simulink model "test_p"  (R2022a)
settings: Solver=FixedStepAuto  StartTime=0.0  StopTime=20  FixedStep=0.005  RelTol=1e-3
values from neighbouring files (symbols this model uses):
  AttDyna_Ixx = 0.0211    [InitParameters.m]
  AttDyna_Iyy = 0.0219    [InitParameters.m]
  AttDyna_Izz = 0.0366    [InitParameters.m]
  ConEfficiency_drone_cM = 1.779e-07    [InitParameters.m]
  ConEfficiency_drone_cT = 1.105e-05    [InitParameters.m]
  ConEfficiency_drone_R = 0.225    [InitParameters.m]
  PowerUnit_CR = 1148    [InitParameters.m]
  PowerUnit_Tm = 0.02    [InitParameters.m]
  PowerUnit_wb = -141.4    [InitParameters.m]
libraries: simulink x53, slpidlib x15, fuzblock x12, mpclib x1
(part 1 of 3)
settings Model: Creator=ZhangZheng  LastModifiedBy=Administrator
settings SolverCC: AlgebraicLoopSolver=TrustRegion
settings DataIOCC: ReturnWorkspaceOutputs=off
settings DebuggingCC: UnconnectedInputMsg=warning  UnconnectedOutputMsg=warning  UnconnectedLineMsg=warning  SFMachineParentedDataDiag=warning  ArithmeticOperatorsInVariantConditions=warning
settings SFSimCC: SimUseLocalCustomCode=off  CustomCodeUndefinedFunction=UseInterfaceOnly
settings RTWCC: RTWUseLocalCustomCode=off

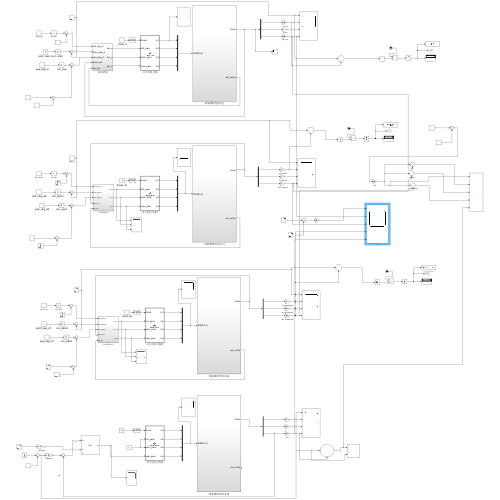
[thumbnail: Simulink's stored preview of the top-level diagram]
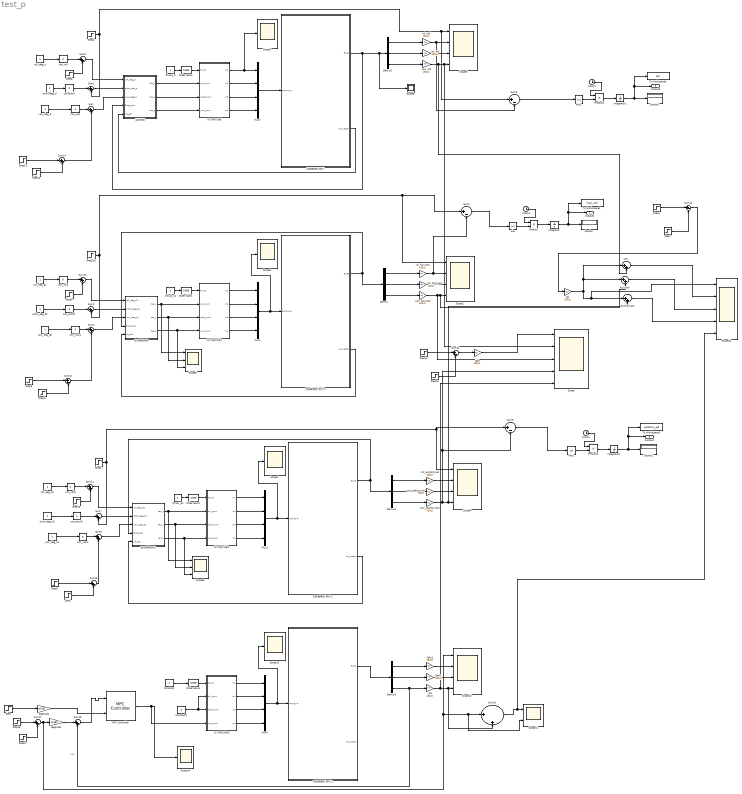
== system test_p ==
  note: sun
  Abs : Abs  SaturateOnIntegerOverflow=off
  Abs1 : Abs  SaturateOnIntegerOverflow=off
  Abs2 : Abs  SaturateOnIntegerOverflow=off
  Clock1 : Clock
      settings: Decimation=20
  Clock2 : Clock
      settings: Decimation=20
  Clock4 : Clock
      settings: Decimation=20
  Constant : Constant
  Constant1 : Constant  Value=0
  Demux{,1..3} (4 alike) : Demux  Outputs=3
  Display : Display
  Display1 : Display
  Display2 : Display
  Gain : Gain  Gain=180/pi
  Gain1 : Gain  Gain=180/pi
  Gain3 : Gain  Gain=180/pi
  Integrator : Integrator
  Integrator1 : Integrator
  Integrator2 : Integrator
  MPC Controller : mpclib/MPC Controller  SCDEnableBlockLinearizationSpecification=on  mpcobj=mpc1  is_multiple=0  enable_value=0  return_u0=off  updateMPCinCallerWorkspace=on  md_inport=off  mv_inport=off  uref_inport=off  return_cost=off  return_mvseq=off  return_qpstatus=off  return_xseq=off  return_state=off  return_ovseq=off  state_inport=off  umin_inport=off  umax_inport=off  ymin_inport=off  ymax_inport=off  cc_inport=off  ywt_inport=off  uwt_inport=off  duwt_inport=off  rhoeps_inport=off  pm_inport=off  MaximumP=10  HorizonChoice=FixedHorizon  n_ts=0.01  n_p=10  n_mv=1  n_md=0  n_ud=0  n_mo=1  n_uo=0  BlockDataType=double  SampleTimeInherited=off  switch_inport=off
  Mux{1..4} (4 alike) : Mux
  Product : Product
  Product1 : Product
  Product2 : Product
  Scope : Scope  NumInputPorts=5
  Scope{1,4,6,12} (4 alike) : Scope  NumInputPorts=4
  Scope10 : Scope  NumInputPorts=5
  Scope11 : Scope  NumInputPorts=2
  Scope{2..3,7,9,13..14} (6 alike) : Scope
  Scope5 : Scope  NumInputPorts=3
  Scope8 : Scope  NumInputPorts=3
  Slider Gain{1..4} (4 alike) : simulink/Math Operations/Slider Gain  gain=0.609  low=0  high=1
  Step : Step  Time=0  After=0  SampleTime=0
  Step1 : Step  Time=8  After=0  SampleTime=0
  Step{2..3,5..6,8..10,13} (8 alike) : Step  Time=5  After=0  SampleTime=0
  Step11 : Step  Time=8  After=0  SampleTime=0
  Step12 : Step  Time=8  After=0  SampleTime=0
  Step14 : Step  Time=5  After=0.05  SampleTime=0
  Step15 : Step  Time=6  After=0.05  SampleTime=0
  Step16 : Step  Time=5  After=2.866  SampleTime=0
  Step17 : Step  Time=6  After=2.866  SampleTime=0
  Step4 : Step  Time=5  After=0.05  SampleTime=0
  Step7 : Step  Time=6  After=0.05  SampleTime=0
  Step_pit : Step  Time=5  After=0  SampleTime=0
  Sum{,1..3,6..7,9..11,18..19} (11 alike) : Sum  Inputs=|++
  Sum{4..5,8,12..17} (9 alike) : Sum  Inputs=|+-
  To Workspace1 : ToWorkspace  VariableName=fuzzy_pid  SaveFormat=Timeseries  SampleTime=-1
  To Workspace2 : ToWorkspace  VariableName=pid  SaveFormat=Timeseries  SampleTime=-1
  To Workspace3 : ToWorkspace  VariableName=psofuzzy_pid  SaveFormat=Timeseries  SampleTime=-1
  con_pitch : simulink/Math Operations/Slider Gain  gain=0  low=-10  high=10
  con_pitch1 : simulink/Math Operations/Slider Gain  gain=0  low=-10  high=10
  con_pitch2 : simulink/Math Operations/Slider Gain  gain=0  low=-10  high=10
  con_roll : simulink/Math Operations/Slider Gain  gain=0  low=-10  high=10
  con_roll1 : simulink/Math Operations/Slider Gain  gain=0  low=-10  high=10
  con_roll2 : simulink/Math Operations/Slider Gain  gain=0  low=-10  high=10
  con_yaw : simulink/Math Operations/Slider Gain  gain=0  low=-10  high=10
  con_yaw1 : simulink/Math Operations/Slider Gain  gain=0  low=-10  high=10
  con_yaw2 : simulink/Math Operations/Slider Gain  gain=0  low=-10  high=10
  deg2rad1 : Gain  Gain=pi/180
  deg2rad2 : Gain  Gain=pi/180
  dis : Gain  Gain=180/pi
  fuzzypid : Sum  Inputs=|++
  pid : Sum  Inputs=|++
  pit_fuzzypid : Gain  Gain=180/pi
  pit_pid : Gain  Gain=180/pi
  pit_psofuzzypid : Gain  Gain=180/pi
  pitch_deg_d : Constant
  pitch_deg_d1 : Constant
  pitch_deg_d2 : Constant
  psofuzzypid : Sum  Inputs=|++
  rol_fuzzypid : Gain  Gain=180/pi
  rol_pid : Gain  Gain=180/pi
  roll_deg_d : Constant
  roll_deg_d1 : Constant
  roll_deg_d2 : Constant
  roll_psofuzzypid : Gain  Gain=180/pi
  thrust_d : Constant
  thrust_d1 : Constant
  thrust_d2 : Constant
  yaw : Gain  Gain=180/pi
  yaw_deg_d : Constant
  yaw_deg_d1 : Constant
  yaw_deg_d2 : Constant
  yaw_fuzzypid : Gain  Gain=180/pi
  yaw_pid : Gain  Gain=180/pi
  yaw_psofuzzypid : Gain  Gain=180/pi
  动力电机分配 : MATLAB Function  TreatAsAtomicUnit=on
  动力电机分配1 : MATLAB Function  TreatAsAtomicUnit=on
  动力电机分配2 : MATLAB Function  TreatAsAtomicUnit=on
  动力电机分配3 : MATLAB Function  TreatAsAtomicUnit=on
  四旋翼模型(简化) : Subsystem
  四旋翼模型(简化)1 : Subsystem
  四旋翼模型(简化)2 : Subsystem
  四旋翼模型(简化)3 : Subsystem
  姿态控制 : Subsystem
  姿态模糊控制 : Subsystem
  姿态模糊控制1 : Subsystem
  Output1 : Outport
  Output3 : Outport  Port=2
  Output2 : Outport  Port=3
  wires:
  动力电机分配/4(m4) -> Mux2/4
  动力电机分配/3(m3) -> Mux2/3
  动力电机分配/2(m2) -> Mux2/2
  动力电机分配/1(m1) -> Scope2/1, Mux2/1
  pitch_deg_d/1 -> con_pitch/1
  Slider Gain3/1 -> 动力电机分配/1(thrust)
  thrust_d/1 -> Slider Gain3/1
  yaw_deg_d/1 -> con_yaw/1
  Mux2/1 -> 四旋翼模型(简化)/1(PWM(1-4))
  姿态控制/1(tao_x) -> 动力电机分配/2(roll_pwm)
  姿态控制/2(tao_y) -> 动力电机分配/3(pitch_pwm)
  姿态控制/3(tao_z) -> 动力电机分配/4(yaw_pwm)
  四旋翼模型(简化)/2(wb_vector) -> 姿态控制/5(wb_act)
  roll_deg_d/1 -> con_roll/1
  con_yaw/1 -> Sum/1
  Sum/1 -> 姿态控制/3(yaw_deg_d)
  con_pitch/1 -> Sum1/1
  Sum1/1 -> 姿态控制/2(pitch_deg_d)
  Step2/1 -> Sum1/2, Sum5/1, Scope6/1
  四旋翼模型(简化)1/1(Euler) -> Demux/1, 姿态模糊控制/4(Euler_act)
  动力电机分配1/3(m3) -> Mux1/3
  动力电机分配1/2(m2) -> Mux1/2
  Slider Gain1/1 -> 动力电机分配1/1(thrust)
  动力电机分配1/4(m4) -> Mux1/4
  Step_pit/1 -> Sum3/2, Scope1/1, Sum4/1
  con_pitch1/1 -> Sum3/1
  Mux1/1 -> Scope3/1, 四旋翼模型(简化)1/1(PWM(1-4))
  Step3/1 -> Sum13/1
  yaw_deg_d2/1 -> con_yaw1/1
  roll_deg_d2/1 -> con_roll1/1
  Sum3/1 -> 姿态模糊控制/2(pitch_deg_d1)
  con_yaw1/1 -> Sum2/1
  动力电机分配1/1(m1) -> Mux1/1
  Sum2/1 -> 姿态模糊控制/3(yaw_deg_d1)
  thrust_d1/1 -> Slider Gain1/1
  四旋翼模型(简化)1/2(wb_vector) -> 姿态模糊控制/5(wb_act)
  pitch_deg_d2/1 -> con_pitch1/1
  姿态模糊控制/1(tao_x) -> Scope5/1, 动力电机分配1/2(roll_pwm)
  姿态模糊控制/2(tao_y) -> Scope5/2, 动力电机分配1/3(pitch_pwm)
  姿态模糊控制/3(tao_z) -> Scope5/3, 动力电机分配1/4(yaw_pwm)
  Demux/1 -> rol_fuzzypid/1
  Demux/3 -> yaw_fuzzypid/1
  Demux/2 -> pit_fuzzypid/1
  rol_fuzzypid/1 -> Sum4/2, Scope1/2
  pit_fuzzypid/1 -> Scope1/3
  yaw_fuzzypid/1 -> Scope/3, fuzzypid/2, Scope1/4
  Demux1/2 -> pit_pid/1
  四旋翼模型(简化)/1(Euler) -> Scope9/1, Demux1/1, 姿态控制/4(Euler_act)
  Demux1/1 -> rol_pid/1
  pit_pid/1 -> Scope6/3
  Demux1/3 -> yaw_pid/1
  rol_pid/1 -> Sum5/2, Scope6/2
  yaw_pid/1 -> pid/2, Scope/2, Scope6/4
  Abs/1 -> Product/2
  Product/1 -> Integrator/1
  Integrator/1 -> Output1/1, To Workspace1/1, Display/1
  Sum4/1 -> Abs/1
  Sum5/1 -> Abs1/1
  姿态模糊控制1/2(tao_y) -> Scope8/2, 动力电机分配2/3(pitch_pwm)
  动力电机分配2/1(m1) -> Mux3/1
  动力电机分配2/2(m2) -> Mux3/2
  yaw_deg_d1/1 -> con_yaw2/1
  pitch_deg_d1/1 -> con_pitch2/1
  thrust_d2/1 -> Slider Gain2/1
  四旋翼模型(简化)2/2(wb_vector) -> 姿态模糊控制1/5(wb_act)
  Demux2/3 -> yaw_psofuzzypid/1
  Demux2/1 -> roll_psofuzzypid/1
  Mux3/1 -> Scope7/1, 四旋翼模型(简化)2/1(PWM(1-4))
  Step6/1 -> Sum7/2, Sum8/1, Scope4/1
  姿态模糊控制1/3(tao_z) -> Scope8/3, 动力电机分配2/4(yaw_pwm)
  四旋翼模型(简化)2/1(Euler) -> Demux2/1, 姿态模糊控制1/4(Euler_act)
  roll_deg_d1/1 -> con_roll2/1
  Sum7/1 -> 姿态模糊控制1/2(pitch_deg_d1)
  pit_psofuzzypid/1 -> Scope4/3
  Slider Gain2/1 -> 动力电机分配2/1(thrust)
  con_pitch2/1 -> Sum7/1
  动力电机分配2/3(m3) -> Mux3/3
  姿态模糊控制1/1(tao_x) -> Scope8/1, 动力电机分配2/2(roll_pwm)
  动力电机分配2/4(m4) -> Mux3/4
  Sum6/1 -> 姿态模糊控制1/3(yaw_deg_d1)
  con_yaw2/1 -> Sum6/1
  Demux2/2 -> pit_psofuzzypid/1
  roll_psofuzzypid/1 -> Scope4/2
  yaw_psofuzzypid/1 -> Sum8/2, Scope/4, psofuzzypid/2, Scope4/4
  Sum8/1 -> Abs2/1
  Clock4/1 -> Product/1
  Step4/1 -> Sum12/1
  Step7/1 -> Sum12/2
  Sum12/1 -> dis/1
  Step8/1 -> Sum9/2
  con_roll/1 -> Sum9/1
  Sum9/1 -> 姿态控制/1(roll_deg_d)
  Step9/1 -> Sum10/2
  con_roll1/1 -> Sum10/1
  Sum10/1 -> 姿态模糊控制/1(roll_deg_d1)
  Step10/1 -> Sum11/2
  con_roll2/1 -> Sum11/1
  Sum11/1 -> 姿态模糊控制1/1(roll_deg_d1)
  dis/1 -> Scope10/1, psofuzzypid/1, fuzzypid/1, pid/1
  Abs1/1 -> Product1/2
  Integrator1/1 -> Output3/1, To Workspace2/1, Display1/1
  Product1/1 -> Integrator1/1
  Clock1/1 -> Product1/1
  Abs2/1 -> Product2/2
  Integrator2/1 -> Output2/1, To Workspace3/1, Display2/1
  Product2/1 -> Integrator2/1
  Clock2/1 -> Product2/1
  Step11/1 -> Sum13/2
  Sum13/1 -> Sum2/2
  Step12/1 -> Sum14/2
  Step13/1 -> Sum14/1
  Sum14/1 -> Sum/2
  Step1/1 -> Sum15/2
  Step5/1 -> Sum15/1
  Sum15/1 -> Sum6/2
  Step14/1 -> Sum16/1
  Step15/1 -> Sum16/2
  Sum16/1 -> Gain/1
  Gain/1 -> Scope/1
  pid/1 -> Scope10/2
  fuzzypid/1 -> Scope10/3
  psofuzzypid/1 -> Scope10/4
  Step17/1 -> Sum17/2
  MPC Controller/1 -> 动力电机分配3/4(yaw_pwm), Scope14/1
  Sum18/1 -> MPC Controller/1
  Sum19/1 -> Scope10/5, Scope11/1
  Step16/1 -> Sum17/1
  deg2rad1/1 -> Sum18/1
  Sum17/1 -> Scope11/2, Sum19/1, Scope12/1, deg2rad1/1
  Mux4/1 -> Scope13/1, 四旋翼模型(简化)3/1(PWM(1-4))
  deg2rad2/1 -> MPC Controller/2
  Demux3/1 -> Gain1/1
  yaw/1 -> Scope/5, Sum19/2, Scope12/4
  Gain1/1 -> Scope12/2
  四旋翼模型(简化)3/1(Euler) -> Demux3/1
  Demux3/3 -> yaw/1, Sum18/2
  动力电机分配3/3(m3) -> Mux4/3
  Constant/1 -> Slider Gain4/1
  Demux3/2 -> Gain3/1
  Step/1 -> deg2rad2/1
  动力电机分配3/4(m4) -> Mux4/4
  Gain3/1 -> Scope12/3
  Slider Gain4/1 -> 动力电机分配3/1(thrust)
  动力电机分配3/2(m2) -> Mux4/2
  动力电机分配3/1(m1) -> Mux4/1
  Constant1/1 -> 动力电机分配3/2(roll_pwm), 动力电机分配3/3(pitch_pwm)

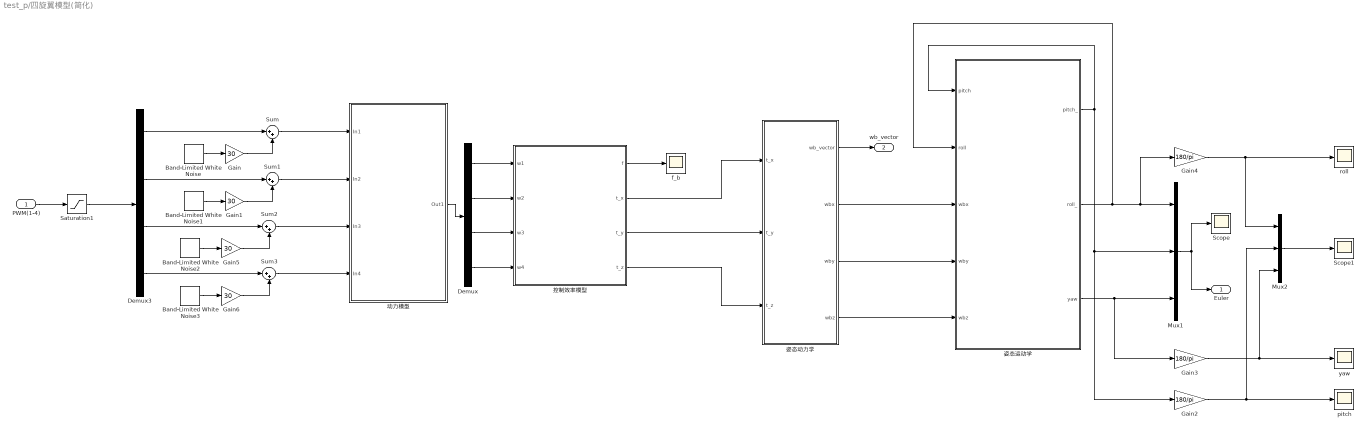
== system test_p/四旋翼模型(简化) ==
  PWM(1-4) : Inport
  Band-Limited White Noise{,1..3} (4 alike) : simulink/Sources/Band-Limited White Noise  Cov=[0.1]  Ts=0.1  seed=[23341]
  Demux : Demux
  Demux3 : Demux
  Gain{,1,5..6} (4 alike) : Gain  Gain=30
  Gain2 : Gain  Gain=180/pi
  Gain3 : Gain  Gain=180/pi
  Gain4 : Gain  Gain=180/pi
  Mux1 : Mux  Inputs=3
  Mux2 : Mux  Inputs=3
  Saturation1 : Saturate  UpperLimit=2000  LowerLimit=1000
  Scope : Scope
  Scope1 : Scope
  Sum{,1..3} (4 alike) : Sum  Inputs=|++
  f_b : Scope
  pitch : Scope
  roll : Scope
  yaw : Scope
  动力模型 : Subsystem
  姿态动力学 : Subsystem
  姿态运动学 : Subsystem
  控制效率模型 : Subsystem
  Euler : Outport  VectorParamsAs1DForOutWhenUnconnected=off
  wb_vector : Outport  Port=2  VectorParamsAs1DForOutWhenUnconnected=off
  wires:
  Saturation1/1 -> Demux3/1
  姿态运动学/1(pitch_) -> Mux1/2, Gain2/1, 姿态运动学/1(pitch)
  Demux/3 -> 控制效率模型/3(w3)
  PWM(1-4)/1 -> Saturation1/1
  控制效率模型/3(t_y) -> 姿态动力学/2(t_y)
  控制效率模型/4(t_z) -> 姿态动力学/3(t_z)
  Demux/2 -> 控制效率模型/2(w2)
  动力模型/1(Out1) -> Demux/1
  Demux/4 -> 控制效率模型/4(w4)
  Demux/1 -> 控制效率模型/1(w1)
  控制效率模型/2(t_x) -> 姿态动力学/1(t_x)
  姿态动力学/2(wbx) -> 姿态运动学/3(wbx)
  姿态运动学/2(roll_) -> Mux1/1, Gain4/1, 姿态运动学/2(roll)
  姿态动力学/1(wb_vector) -> wb_vector/1
  姿态运动学/3(yaw) -> Mux1/3, Gain3/1
  姿态动力学/4(wbz) -> 姿态运动学/5(wbz)
  姿态动力学/3(wby) -> 姿态运动学/4(wby)
  Mux1/1 -> Euler/1, Scope/1
  Mux2/1 -> Scope1/1
  Gain4/1 -> Mux2/1, roll/1
  Gain2/1 -> pitch/1, Mux2/2
  Gain3/1 -> yaw/1, Mux2/3
  控制效率模型/1(f) -> f_b/1
  Band-Limited White Noise/1 -> Gain/1
  Band-Limited White Noise1/1 -> Gain1/1
  Sum3/1 -> 动力模型/4(In4)
  Demux3/1 -> Sum/1
  Sum2/1 -> 动力模型/3(In3)
  Demux3/3 -> Sum2/1
  Demux3/4 -> Sum3/1
  Band-Limited White Noise3/1 -> Gain6/1
  Gain5/1 -> Sum2/2
  Gain6/1 -> Sum3/2
  Gain1/1 -> Sum1/2
  Sum1/1 -> 动力模型/2(In2)
  Sum/1 -> 动力模型/1(In1)
  Demux3/2 -> Sum1/1
  Gain/1 -> Sum/2
  Band-Limited White Noise2/1 -> Gain5/1

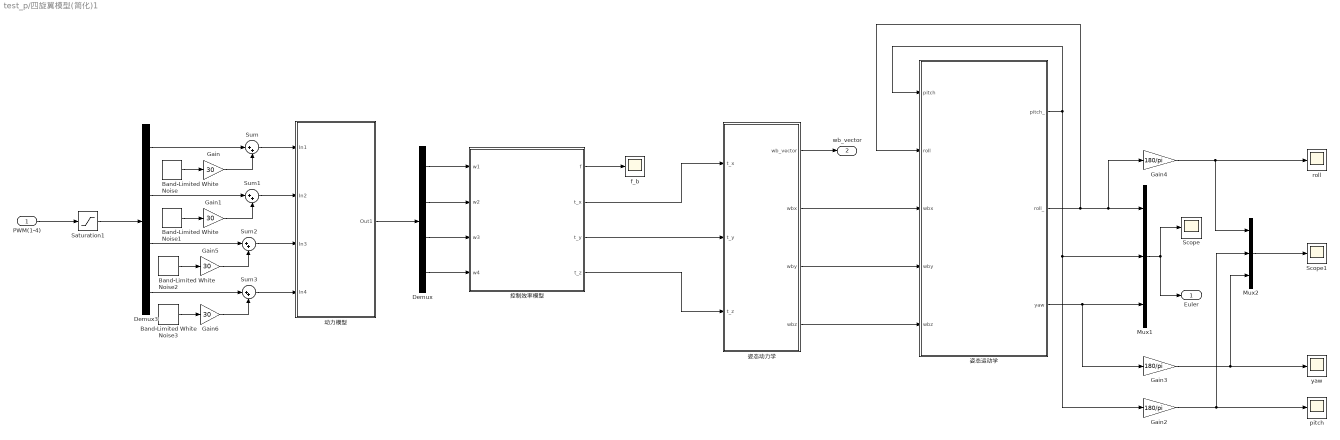
== system test_p/四旋翼模型(简化)1 ==
  PWM(1-4) : Inport
  Band-Limited White Noise{,1..3} (4 alike) : simulink/Sources/Band-Limited White Noise  Cov=[0.1]  Ts=0.1  seed=[23341]
  Demux : Demux
  Demux3 : Demux
  Gain{,1,5..6} (4 alike) : Gain  Gain=30
  Gain2 : Gain  Gain=180/pi
  Gain3 : Gain  Gain=180/pi
  Gain4 : Gain  Gain=180/pi
  Mux1 : Mux  Inputs=3
  Mux2 : Mux  Inputs=3
  Saturation1 : Saturate  UpperLimit=2000  LowerLimit=1000
  Scope : Scope
  Scope1 : Scope
  Sum{,1..3} (4 alike) : Sum  Inputs=|++
  f_b : Scope
  pitch : Scope
  roll : Scope
  yaw : Scope
  动力模型 : Subsystem
  姿态动力学 : Subsystem
  姿态运动学 : Subsystem
  控制效率模型 : Subsystem
  Euler : Outport  VectorParamsAs1DForOutWhenUnconnected=off
  wb_vector : Outport  Port=2  VectorParamsAs1DForOutWhenUnconnected=off
  wires:
  Saturation1/1 -> Demux3/1
  姿态运动学/1(pitch_) -> Mux1/2, Gain2/1, 姿态运动学/1(pitch)
  Demux/3 -> 控制效率模型/3(w3)
  PWM(1-4)/1 -> Saturation1/1
  控制效率模型/3(t_y) -> 姿态动力学/2(t_y)
  控制效率模型/4(t_z) -> 姿态动力学/3(t_z)
  Demux/2 -> 控制效率模型/2(w2)
  动力模型/1(Out1) -> Demux/1
  Demux/4 -> 控制效率模型/4(w4)
  Demux/1 -> 控制效率模型/1(w1)
  控制效率模型/2(t_x) -> 姿态动力学/1(t_x)
  姿态动力学/2(wbx) -> 姿态运动学/3(wbx)
  姿态运动学/2(roll_) -> Mux1/1, Gain4/1, 姿态运动学/2(roll)
  姿态动力学/1(wb_vector) -> wb_vector/1
  姿态运动学/3(yaw) -> Mux1/3, Gain3/1
  姿态动力学/4(wbz) -> 姿态运动学/5(wbz)
  姿态动力学/3(wby) -> 姿态运动学/4(wby)
  Mux1/1 -> Euler/1, Scope/1
  Mux2/1 -> Scope1/1
  Gain4/1 -> Mux2/1, roll/1
  Gain2/1 -> pitch/1, Mux2/2
  Gain3/1 -> yaw/1, Mux2/3
  控制效率模型/1(f) -> f_b/1
  Band-Limited White Noise/1 -> Gain/1
  Gain/1 -> Sum/2
  Demux3/1 -> Sum/1
  Sum/1 -> 动力模型/1(In1)
  Demux3/2 -> Sum1/1
  Gain1/1 -> Sum1/2
  Band-Limited White Noise1/1 -> Gain1/1
  Sum1/1 -> 动力模型/2(In2)
  Demux3/3 -> Sum2/1
  Gain5/1 -> Sum2/2
  Band-Limited White Noise2/1 -> Gain5/1
  Sum2/1 -> 动力模型/3(In3)
  Demux3/4 -> Sum3/1
  Gain6/1 -> Sum3/2
  Band-Limited White Noise3/1 -> Gain6/1
  Sum3/1 -> 动力模型/4(In4)

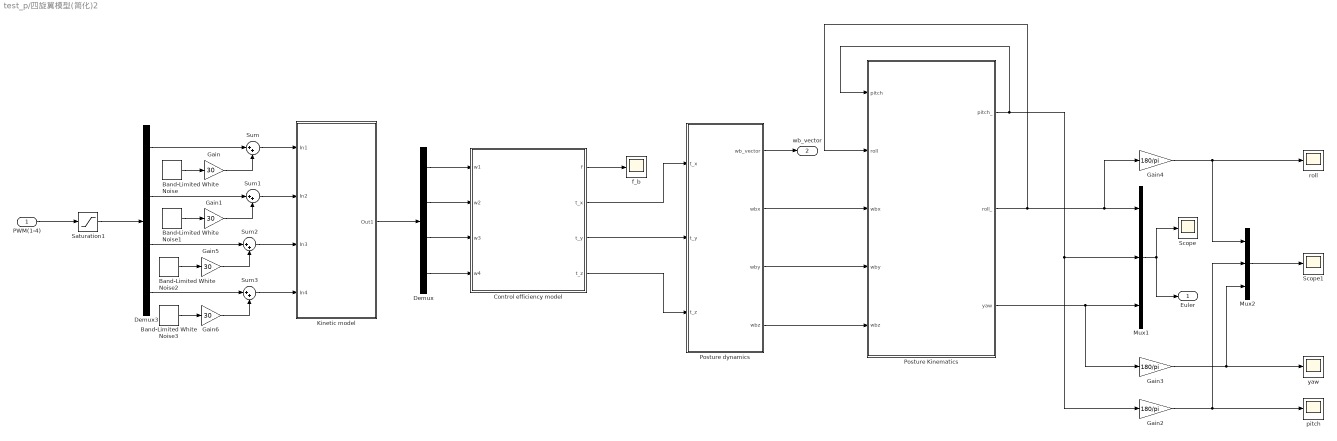
== system test_p/四旋翼模型(简化)2 ==
  PWM(1-4) : Inport
  Band-Limited White Noise{,1..3} (4 alike) : simulink/Sources/Band-Limited White Noise  Cov=[0.1]  Ts=0.1  seed=[23341]
  Control efficiency model : Subsystem
  Demux : Demux
  Demux3 : Demux
  Gain{,1,5..6} (4 alike) : Gain  Gain=30
  Gain2 : Gain  Gain=180/pi
  Gain3 : Gain  Gain=180/pi
  Gain4 : Gain  Gain=180/pi
  Kinetic model : Subsystem
  Mux1 : Mux  Inputs=3
  Mux2 : Mux  Inputs=3
  Posture Kinematics : Subsystem
  Posture dynamics : Subsystem
  Saturation1 : Saturate  UpperLimit=2000  LowerLimit=1000
  Scope : Scope
  Scope1 : Scope
  Sum{,1..3} (4 alike) : Sum  Inputs=|++
  f_b : Scope
  pitch : Scope
  roll : Scope
  yaw : Scope
  Euler : Outport  VectorParamsAs1DForOutWhenUnconnected=off
  wb_vector : Outport  Port=2  VectorParamsAs1DForOutWhenUnconnected=off
  wires:
  Saturation1/1 -> Demux3/1
  Posture Kinematics/1(pitch_) -> Mux1/2, Gain2/1, Posture Kinematics/1(pitch)
  Demux/3 -> Control efficiency model/3(w3)
  PWM(1-4)/1 -> Saturation1/1
  Control efficiency model/3(t_y) -> Posture dynamics/2(t_y)
  Control efficiency model/4(t_z) -> Posture dynamics/3(t_z)
  Demux/2 -> Control efficiency model/2(w2)
  Kinetic model/1(Out1) -> Demux/1
  Demux/4 -> Control efficiency model/4(w4)
  Demux/1 -> Control efficiency model/1(w1)
  Control efficiency model/2(t_x) -> Posture dynamics/1(t_x)
  Posture dynamics/2(wbx) -> Posture Kinematics/3(wbx)
  Posture Kinematics/2(roll_) -> Mux1/1, Gain4/1, Posture Kinematics/2(roll)
  Posture dynamics/1(wb_vector) -> wb_vector/1
  Posture Kinematics/3(yaw) -> Mux1/3, Gain3/1
  Posture dynamics/4(wbz) -> Posture Kinematics/5(wbz)
  Posture dynamics/3(wby) -> Posture Kinematics/4(wby)
  Mux1/1 -> Euler/1, Scope/1
  Mux2/1 -> Scope1/1
  Gain4/1 -> Mux2/1, roll/1
  Gain2/1 -> pitch/1, Mux2/2
  Gain3/1 -> yaw/1, Mux2/3
  Control efficiency model/1(f) -> f_b/1
  Band-Limited White Noise/1 -> Gain/1
  Gain/1 -> Sum/2
  Demux3/1 -> Sum/1
  Sum/1 -> Kinetic model/1(In1)
  Demux3/2 -> Sum1/1
  Gain1/1 -> Sum1/2
  Band-Limited White Noise1/1 -> Gain1/1
  Sum1/1 -> Kinetic model/2(In2)
  Demux3/3 -> Sum2/1
  Gain5/1 -> Sum2/2
  Band-Limited White Noise2/1 -> Gain5/1
  Sum2/1 -> Kinetic model/3(In3)
  Demux3/4 -> Sum3/1
  Gain6/1 -> Sum3/2
  Band-Limited White Noise3/1 -> Gain6/1
  Sum3/1 -> Kinetic model/4(In4)

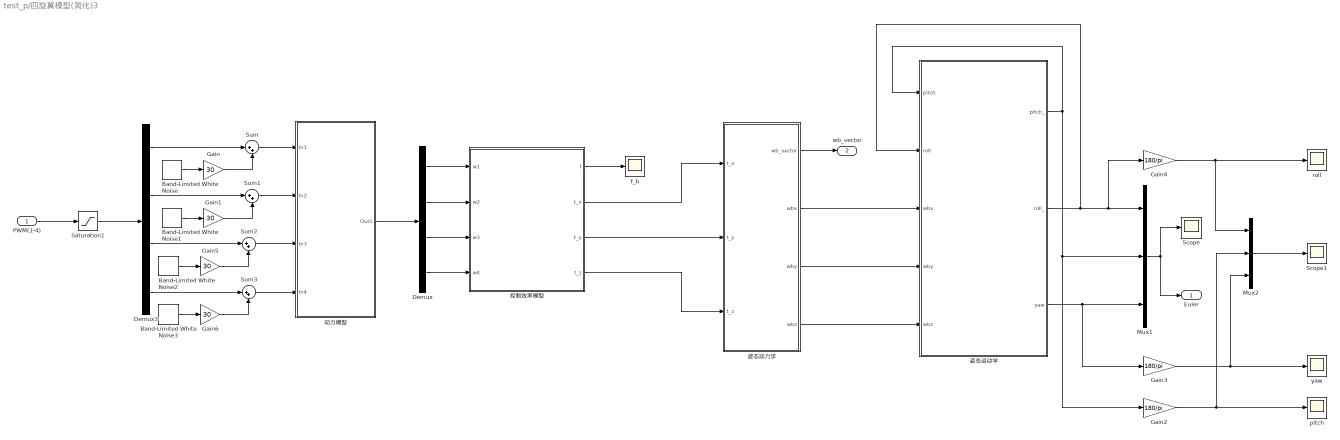
== system test_p/四旋翼模型(简化)3 ==
  PWM(1-4) : Inport
  Band-Limited White Noise{,1..3} (4 alike) : simulink/Sources/Band-Limited White Noise  Cov=[0.1]  Ts=0.1  seed=[23341]
  Demux : Demux
  Demux3 : Demux
  Gain{,1,5..6} (4 alike) : Gain  Gain=30
  Gain2 : Gain  Gain=180/pi
  Gain3 : Gain  Gain=180/pi
  Gain4 : Gain  Gain=180/pi
  Mux1 : Mux  Inputs=3
  Mux2 : Mux  Inputs=3
  Saturation1 : Saturate  UpperLimit=2000  LowerLimit=1000
  Scope : Scope
  Scope1 : Scope
  Sum{,1..3} (4 alike) : Sum  Inputs=|++
  f_b : Scope
  pitch : Scope
  roll : Scope
  yaw : Scope
  动力模型 : Subsystem
  姿态动力学 : Subsystem
  姿态运动学 : Subsystem
  控制效率模型 : Subsystem
  Euler : Outport  VectorParamsAs1DForOutWhenUnconnected=off
  wb_vector : Outport  Port=2  VectorParamsAs1DForOutWhenUnconnected=off
  wires:
  Saturation1/1 -> Demux3/1
  姿态运动学/1(pitch_) -> Mux1/2, Gain2/1, 姿态运动学/1(pitch)
  Demux/3 -> 控制效率模型/3(w3)
  PWM(1-4)/1 -> Saturation1/1
  控制效率模型/3(t_y) -> 姿态动力学/2(t_y)
  控制效率模型/4(t_z) -> 姿态动力学/3(t_z)
  Demux/2 -> 控制效率模型/2(w2)
  动力模型/1(Out1) -> Demux/1
  Demux/4 -> 控制效率模型/4(w4)
  Demux/1 -> 控制效率模型/1(w1)
  控制效率模型/2(t_x) -> 姿态动力学/1(t_x)
  姿态动力学/2(wbx) -> 姿态运动学/3(wbx)
  姿态运动学/2(roll_) -> Mux1/1, Gain4/1, 姿态运动学/2(roll)
  姿态动力学/1(wb_vector) -> wb_vector/1
  姿态运动学/3(yaw) -> Mux1/3, Gain3/1
  姿态动力学/4(wbz) -> 姿态运动学/5(wbz)
  姿态动力学/3(wby) -> 姿态运动学/4(wby)
  Mux1/1 -> Euler/1, Scope/1
  Mux2/1 -> Scope1/1
  Gain4/1 -> Mux2/1, roll/1
  Gain2/1 -> pitch/1, Mux2/2
  Gain3/1 -> yaw/1, Mux2/3
  控制效率模型/1(f) -> f_b/1
  Band-Limited White Noise/1 -> Gain/1
  Gain/1 -> Sum/2
  Demux3/1 -> Sum/1
  Sum/1 -> 动力模型/1(In1)
  Demux3/2 -> Sum1/1
  Gain1/1 -> Sum1/2
  Band-Limited White Noise1/1 -> Gain1/1
  Sum1/1 -> 动力模型/2(In2)
  Demux3/3 -> Sum2/1
  Gain5/1 -> Sum2/2
  Band-Limited White Noise2/1 -> Gain5/1
  Sum2/1 -> 动力模型/3(In3)
  Demux3/4 -> Sum3/1
  Gain6/1 -> Sum3/2
  Band-Limited White Noise3/1 -> Gain6/1
  Sum3/1 -> 动力模型/4(In4)

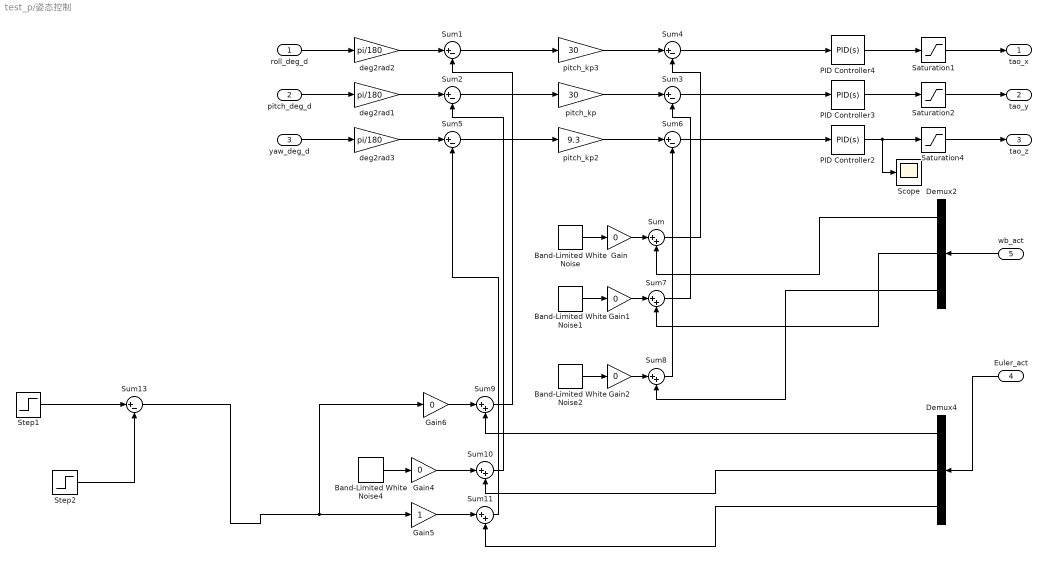
== system test_p/姿态控制 ==
  roll_deg_d : Inport
  pitch_deg_d : Inport  Port=2
  yaw_deg_d : Inport  Port=3
  Euler_act : Inport  Port=4
  wb_act : Inport  Port=5
  Band-Limited White Noise{,1..2,4} (4 alike) : simulink/Sources/Band-Limited White Noise  Cov=[0.1]  Ts=0.1  seed=[23341]
  Demux2 : Demux  Outputs=3
  Demux4 : Demux  Outputs=3
  Gain{,1..2,4,6} (5 alike) : Gain  Gain=0
  Gain5 : Gain
  PID Controller2 : slpidlib/PID Controller  Controller=PID  Form=Parallel  TimeDomain=Continuous-time  UseExternalTs=off  SampleTime=-1  IntegratorMethod=Forward Euler  FilterMethod=Forward Euler  ControllerParametersSource=internal  P=34  I=0  UseKiTs=off  D=0.1  N=100  UseFilter=on  TunerSelectOption=Transfer Function Based (PID Tuner App)  InitialConditionSource=internal  InitialConditionForIntegrator=0  InitialConditionForFilter=0  DifferentiatorICPrevScaledInput=0  ExternalReset=none  TrackingMode=off  Kt=1  LimitOutput=off  SatLimitsSource=internal  UpperSaturationLimit=inf  LowerSaturationLimit=-inf  LinearizeAsGain=on  AntiWindupMode=none  Kb=1  POutMin=[]  POutMax=[]  IOutMin=[]  IOutMax=[]  DOutMin=[]  DOutMax=[]  NOutMin=[]  NOutMax=[]  SumOutMin=[]  SumOutMax=[]  SaturationOutMin=[]  SaturationOutMax=[]  PParamMin=[]  PParamMax=[]  IParamMin=[]  IParamMax=[]  DParamMin=[]  DParamMax=[]  NParamMin=[]  NParamMax=[]  KbParamMin=[]  KbParamMax=[]  KtParamMin=[]  KtParamMax=[]  KbOutMin=[]  KbOutMax=[]  KtOutMin=[]  KtOutMax=[]  IntegratorOutMin=[]  IntegratorOutMax=[]  FilterOutMin=[]  FilterOutMax=[]  SumI1OutMin=[]  SumI1OutMax=[]  SumI2OutMin=[]  SumI2OutMax=[]  SumI3OutMin=[]  SumI3OutMax=[]  SumI4OutMin=[]  SumI4OutMax=[]  SumDOutMin=[]  SumDOutMax=[]  DifferentiatorOutMin=[]  DifferentiatorOutMax=[]  FilterDiffOutCoefMin=[]  FilterDiffOutCoefMax=[]  ReciprocalOutMin=[]  ReciprocalOutMax=[]  SumDenOutMin=[]  SumDenOutMax=[]  SumNumOutMin=[]  SumNumOutMax=[]  DivideOutMin=[]  DivideOutMax=[]  UdiffTsProdOutMin=[]  UdiffTsProdOutMax=[]  NTsProdOutMin=[]  NTsProdOutMax=[]  UintegralTsProdOutMin=[]  UintegralTsProdOutMax=[]  UngainTsProdOutMin=[]  UngainTsProdOutMax=[]  ClampingZeroOutDataTypeStr=Inherit: Inherit via back propagation  ClampingZeroOutMin=[]  ClampingZeroOutMax=[]  FilterDenConstantOutDataTypeStr=Inherit: Inherit via back propagation  FilterDenConstantOutMin=[]  FilterDenConstantOutMax=[]  PCopyOutDataTypeStr=Inherit: Inherit via back propagation  PCopyOutMin=[]  PCopyOutMax=[]  NCopyOutDataTypeStr=Inherit: Inherit via back propagation  NCopyOutMin=[]  NCopyOutMax=[]  IntegratorContinuousStateAttributes=''  IntegratorStateMustResolveToSignalObject=off  IntegratorRTWStateStorageClass=Auto  FilterContinuousStateAttributes=''  FilterStateMustResolveToSignalObject=off  FilterRTWStateStorageClass=Auto  ParallelPVariant=InternalParameters  IdealPVariant=Disabled  IVariant=InternalParameters  DVariant=InternalParameters  IntegratorVariant=Continuous  SatVariant=Disabled  AWVariant=Passthrough  PCopyVariant=Disabled  TRVariant=Disabled  FdbkBlocksVariant=Forward  IdealPFdbkVariant=Disabled  SatFdbkVariant=Disabled  DerivativeFilterVariant=ContFilter  NVariant=InternalParameters  NCopyVariant=Disabled  FilterICVariant=InternalICsFilter  IntegratorICVariant=InternalICs  ExternalResetVariant=Disabled  TRSumVariant=Passthrough  SumFdbkVariant=Disabled  SumVariant=Sum_PID  TsampFilterVariant=InternalTs  TsampNgainVariant=Passthrough  TsampIntegralVariant=Passthrough  ExternalSaturationOutDataTypeStr=Inherit: Same as second input  aMode=0
  PID Controller3 : slpidlib/PID Controller  Controller=PID  Form=Parallel  TimeDomain=Continuous-time  UseExternalTs=off  SampleTime=-1  IntegratorMethod=Forward Euler  FilterMethod=Forward Euler  ControllerParametersSource=internal  P=0.3  I=1.4  UseKiTs=off  D=0.01  N=100  UseFilter=on  TunerSelectOption=Transfer Function Based (PID Tuner App)  InitialConditionSource=internal  InitialConditionForIntegrator=0  InitialConditionForFilter=0  DifferentiatorICPrevScaledInput=0  ExternalReset=none  TrackingMode=off  Kt=1  LimitOutput=off  SatLimitsSource=internal  UpperSaturationLimit=inf  LowerSaturationLimit=-inf  LinearizeAsGain=on  AntiWindupMode=none  Kb=1  POutMin=[]  POutMax=[]  IOutMin=[]  IOutMax=[]  DOutMin=[]  DOutMax=[]  NOutMin=[]  NOutMax=[]  SumOutMin=[]  SumOutMax=[]  SaturationOutMin=[]  SaturationOutMax=[]  PParamMin=[]  PParamMax=[]  IParamMin=[]  IParamMax=[]  DParamMin=[]  DParamMax=[]  NParamMin=[]  NParamMax=[]  KbParamMin=[]  KbParamMax=[]  KtParamMin=[]  KtParamMax=[]  KbOutMin=[]  KbOutMax=[]  KtOutMin=[]  KtOutMax=[]  IntegratorOutMin=[]  IntegratorOutMax=[]  FilterOutMin=[]  FilterOutMax=[]  SumI1OutMin=[]  SumI1OutMax=[]  SumI2OutMin=[]  SumI2OutMax=[]  SumI3OutMin=[]  SumI3OutMax=[]  SumI4OutMin=[]  SumI4OutMax=[]  SumDOutMin=[]  SumDOutMax=[]  DifferentiatorOutMin=[]  DifferentiatorOutMax=[]  FilterDiffOutCoefMin=[]  FilterDiffOutCoefMax=[]  ReciprocalOutMin=[]  ReciprocalOutMax=[]  SumDenOutMin=[]  SumDenOutMax=[]  SumNumOutMin=[]  SumNumOutMax=[]  DivideOutMin=[]  DivideOutMax=[]  UdiffTsProdOutMin=[]  UdiffTsProdOutMax=[]  NTsProdOutMin=[]  NTsProdOutMax=[]  UintegralTsProdOutMin=[]  UintegralTsProdOutMax=[]  UngainTsProdOutMin=[]  UngainTsProdOutMax=[]  ClampingZeroOutDataTypeStr=Inherit: Inherit via back propagation  ClampingZeroOutMin=[]  ClampingZeroOutMax=[]  FilterDenConstantOutDataTypeStr=Inherit: Inherit via back propagation  FilterDenConstantOutMin=[]  FilterDenConstantOutMax=[]  PCopyOutDataTypeStr=Inherit: Inherit via back propagation  PCopyOutMin=[]  PCopyOutMax=[]  NCopyOutDataTypeStr=Inherit: Inherit via back propagation  NCopyOutMin=[]  NCopyOutMax=[]  IntegratorContinuousStateAttributes=''  IntegratorStateMustResolveToSignalObject=off  IntegratorRTWStateStorageClass=Auto  FilterContinuousStateAttributes=''  FilterStateMustResolveToSignalObject=off  FilterRTWStateStorageClass=Auto  ParallelPVariant=InternalParameters  IdealPVariant=Disabled  IVariant=InternalParameters  DVariant=InternalParameters  IntegratorVariant=Continuous  SatVariant=Disabled  AWVariant=Passthrough  PCopyVariant=Disabled  TRVariant=Disabled  FdbkBlocksVariant=Forward  IdealPFdbkVariant=Disabled  SatFdbkVariant=Disabled  DerivativeFilterVariant=ContFilter  NVariant=InternalParameters  NCopyVariant=Disabled  FilterICVariant=InternalICsFilter  IntegratorICVariant=InternalICs  ExternalResetVariant=Disabled  TRSumVariant=Passthrough  SumFdbkVariant=Disabled  SumVariant=Sum_PID  TsampFilterVariant=InternalTs  TsampNgainVariant=Passthrough  TsampIntegralVariant=Passthrough  ExternalSaturationOutDataTypeStr=Inherit: Same as second input  aMode=0
  PID Controller4 : slpidlib/PID Controller  Controller=PID  Form=Parallel  TimeDomain=Continuous-time  UseExternalTs=off  SampleTime=-1  IntegratorMethod=Forward Euler  FilterMethod=Forward Euler  ControllerParametersSource=internal  P=0.3  I=1.4  UseKiTs=off  D=0.01  N=100  UseFilter=on  TunerSelectOption=Transfer Function Based (PID Tuner App)  InitialConditionSource=internal  InitialConditionForIntegrator=0  InitialConditionForFilter=0  DifferentiatorICPrevScaledInput=0  ExternalReset=none  TrackingMode=off  Kt=1  LimitOutput=off  SatLimitsSource=internal  UpperSaturationLimit=inf  LowerSaturationLimit=-inf  LinearizeAsGain=on  AntiWindupMode=none  Kb=1  POutMin=[]  POutMax=[]  IOutMin=[]  IOutMax=[]  DOutMin=[]  DOutMax=[]  NOutMin=[]  NOutMax=[]  SumOutMin=[]  SumOutMax=[]  SaturationOutMin=[]  SaturationOutMax=[]  PParamMin=[]  PParamMax=[]  IParamMin=[]  IParamMax=[]  DParamMin=[]  DParamMax=[]  NParamMin=[]  NParamMax=[]  KbParamMin=[]  KbParamMax=[]  KtParamMin=[]  KtParamMax=[]  KbOutMin=[]  KbOutMax=[]  KtOutMin=[]  KtOutMax=[]  IntegratorOutMin=[]  IntegratorOutMax=[]  FilterOutMin=[]  FilterOutMax=[]  SumI1OutMin=[]  SumI1OutMax=[]  SumI2OutMin=[]  SumI2OutMax=[]  SumI3OutMin=[]  SumI3OutMax=[]  SumI4OutMin=[]  SumI4OutMax=[]  SumDOutMin=[]  SumDOutMax=[]  DifferentiatorOutMin=[]  DifferentiatorOutMax=[]  FilterDiffOutCoefMin=[]  FilterDiffOutCoefMax=[]  ReciprocalOutMin=[]  ReciprocalOutMax=[]  SumDenOutMin=[]  SumDenOutMax=[]  SumNumOutMin=[]  SumNumOutMax=[]  DivideOutMin=[]  DivideOutMax=[]  UdiffTsProdOutMin=[]  UdiffTsProdOutMax=[]  NTsProdOutMin=[]  NTsProdOutMax=[]  UintegralTsProdOutMin=[]  UintegralTsProdOutMax=[]  UngainTsProdOutMin=[]  UngainTsProdOutMax=[]  ClampingZeroOutDataTypeStr=Inherit: Inherit via back propagation  ClampingZeroOutMin=[]  ClampingZeroOutMax=[]  FilterDenConstantOutDataTypeStr=Inherit: Inherit via back propagation  FilterDenConstantOutMin=[]  FilterDenConstantOutMax=[]  PCopyOutDataTypeStr=Inherit: Inherit via back propagation  PCopyOutMin=[]  PCopyOutMax=[]  NCopyOutDataTypeStr=Inherit: Inherit via back propagation  NCopyOutMin=[]  NCopyOutMax=[]  IntegratorContinuousStateAttributes=''  IntegratorStateMustResolveToSignalObject=off  IntegratorRTWStateStorageClass=Auto  FilterContinuousStateAttributes=''  FilterStateMustResolveToSignalObject=off  FilterRTWStateStorageClass=Auto  ParallelPVariant=InternalParameters  IdealPVariant=Disabled  IVariant=InternalParameters  DVariant=InternalParameters  IntegratorVariant=Continuous  SatVariant=Disabled  AWVariant=Passthrough  PCopyVariant=Disabled  TRVariant=Disabled  FdbkBlocksVariant=Forward  IdealPFdbkVariant=Disabled  SatFdbkVariant=Disabled  DerivativeFilterVariant=ContFilter  NVariant=InternalParameters  NCopyVariant=Disabled  FilterICVariant=InternalICsFilter  IntegratorICVariant=InternalICs  ExternalResetVariant=Disabled  TRSumVariant=Passthrough  SumFdbkVariant=Disabled  SumVariant=Sum_PID  TsampFilterVariant=InternalTs  TsampNgainVariant=Passthrough  TsampIntegralVariant=Passthrough  ExternalSaturationOutDataTypeStr=Inherit: Same as second input  aMode=0
  Saturation1 : Saturate  UpperLimit=1  LowerLimit=-1
  Saturation2 : Saturate  UpperLimit=1  LowerLimit=-1
  Saturation4 : Saturate  UpperLimit=1  LowerLimit=-1
  Scope : Scope
  Step1 : Step  Time=5  After=0.05  SampleTime=0
  Step2 : Step  Time=6  After=0.05  SampleTime=0
  Sum{,7..11} (6 alike) : Sum  Inputs=|++
  Sum{1..6,13} (7 alike) : Sum  Inputs=|+-
  deg2rad1 : Gain  Gain=pi/180
  deg2rad2 : Gain  Gain=pi/180
  deg2rad3 : Gain  Gain=pi/180
  pitch_kp : Gain  Gain=30
  pitch_kp2 : Gain  Gain=9.3
  pitch_kp3 : Gain  Gain=30
  tao_x : Outport  VectorParamsAs1DForOutWhenUnconnected=off
  tao_y : Outport  Port=2  VectorParamsAs1DForOutWhenUnconnected=off
  tao_z : Outport  Port=3  VectorParamsAs1DForOutWhenUnconnected=off
  wires:
  roll_deg_d/1 -> deg2rad2/1
  pitch_deg_d/1 -> deg2rad1/1
  Sum3/1 -> PID Controller3/1
  Saturation2/1 -> tao_y/1
  Sum2/1 -> pitch_kp/1
  PID Controller3/1 -> Saturation2/1
  deg2rad1/1 -> Sum2/1
  Sum1/1 -> pitch_kp3/1
  Saturation4/1 -> tao_z/1
  pitch_kp2/1 -> Sum6/1
  pitch_kp/1 -> Sum3/1
  deg2rad2/1 -> Sum1/1
  wb_act/1 -> Demux2/1
  PID Controller2/1 -> Scope/1, Saturation4/1
  yaw_deg_d/1 -> deg2rad3/1
  deg2rad3/1 -> Sum5/1
  Sum5/1 -> pitch_kp2/1
  Sum6/1 -> PID Controller2/1
  Euler_act/1 -> Demux4/1
  Saturation1/1 -> tao_x/1
  PID Controller4/1 -> Saturation1/1
  pitch_kp3/1 -> Sum4/1
  Sum4/1 -> PID Controller4/1
  Gain/1 -> Sum/1
  Band-Limited White Noise/1 -> Gain/1
  Demux2/1 -> Sum/2
  Sum/1 -> Sum4/2
  Gain1/1 -> Sum7/1
  Band-Limited White Noise1/1 -> Gain1/1
  Demux2/2 -> Sum7/2
  Sum7/1 -> Sum3/2
  Gain2/1 -> Sum8/1
  Band-Limited White Noise2/1 -> Gain2/1
  Demux2/3 -> Sum8/2
  Sum8/1 -> Sum6/2
  Demux4/1 -> Sum9/2
  Sum9/1 -> Sum1/2
  Band-Limited White Noise4/1 -> Gain4/1
  Gain4/1 -> Sum10/1
  Demux4/2 -> Sum10/2
  Sum10/1 -> Sum2/2
  Sum13/1 -> Gain6/1, Gain5/1
  Gain5/1 -> Sum11/1
  Demux4/3 -> Sum11/2
  Sum11/1 -> Sum5/2
  Gain6/1 -> Sum9/1
  Step2/1 -> Sum13/2
  Step1/1 -> Sum13/1
